simulink model "simulink_model_GT"  (R2024b)
settings: Solver=VariableStepAuto  StartTime=0.0  StopTime=10.0  RelTol=1e-3
undefined symbols (not defined in the file): DiscIntNeverNeededParam
settings Model: Creator=xinxing  LastModifiedBy=xinxing

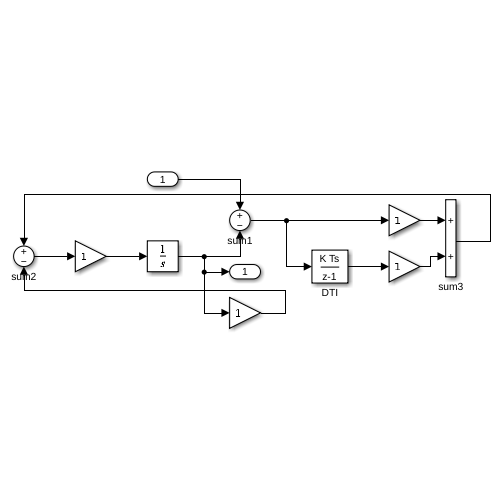
[thumbnail: Simulink's stored preview of the top-level diagram]
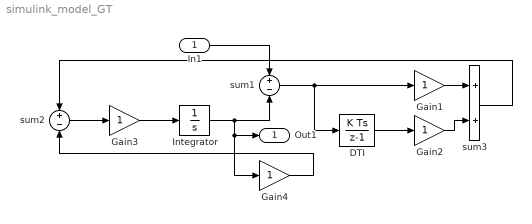
== system simulink_model_GT ==
  In1 : Inport
  DTI : DiscreteIntegrator  SampleTime=-1  ICPrevOutput=DiscIntNeverNeededParam  ICPrevScaledInput=DiscIntNeverNeededParam
  Gain{1..4} (4 alike) : Gain
  Integrator : Integrator
  sum1 : Sum  Inputs=+-
  sum2 : Sum  Inputs=+-
  sum3 : Sum
  Out1 : Outport
  wires:
  Gain2/1 -> sum3/2
  Gain1/1 -> sum3/1
  DTI/1 -> Gain2/1
  Gain4/1 -> sum2/2
  Integrator/1 -> Gain4/1, Out1/1, sum1/2
  sum1/1 -> DTI/1, Gain1/1
  In1/1 -> sum1/1
  sum3/1 -> sum2/1
  Gain3/1 -> Integrator/1
  sum2/1 -> Gain3/1
